simulink model "PendulumSimulation"  (R2020b)
settings: Solver=VariableStepAuto  StartTime=0.0  StopTime=T  RelTol=1e-3
values from neighbouring files (symbols this model uses):
  K = place(A', C', [-5,-2])'./d    [DifferentiatorParameter.m]    (also in Observer_parameter.m = lqr(A, B, eye(4), 10); Project.m = lqr(A, B, eye(4), 2))
  pendulumParameter = PendulumParameter()    [Project.m]
  T = 10    [DifferentiatorParameter.m]    (also in Observer_parameter.m; Project.m)
  Te = 1e-3    (= 0.001)    [DifferentiatorParameter.m]    (also in Observer_parameter.m; Project.m)
  X_eq = [0;pi;0;0]    [Observer_parameter.m]    (also in Project.m = [0;-pi;0;0])
undefined symbols (not defined in the file or in its folder): sigbuilder_block
libraries: simulink_extras x1, vrlib x1
settings Model: Creator=vorps  LastModifiedBy=vorps
settings SolverCC: ZeroCrossAlgorithm=Adaptive
settings DebuggingCC: IgnoredZcDiagnostic=none

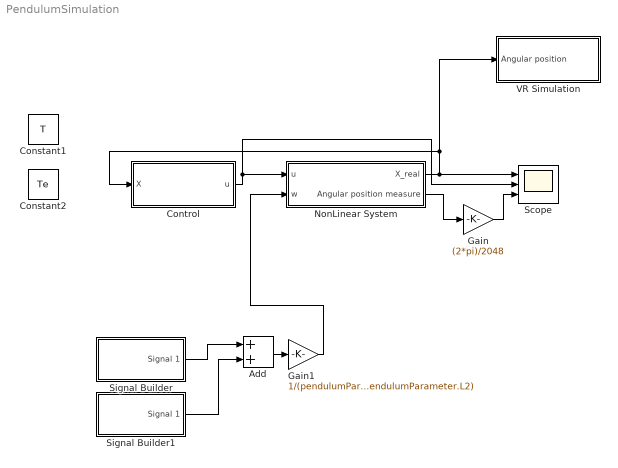
== system PendulumSimulation ==
  Add : Sum
  Constant1 : Constant  Value=T
  Constant2 : Constant  Value=Te
  Control : Subsystem
  Gain : Gain  Gain=(2*pi)/2048
  Gain1 : Gain  Gain=1/(pendulumParameter.M2*pendulumParameter.L2)
  NonLinear System : Subsystem
  Scope : Scope  NumInputPorts=3
  Signal Builder : Subsystem  Tag=STV Subsys  LoadFcn=sigbuilder_block('load');  StartFcn=sigbuilder_block('start');  StopFcn=sigbuilder_block('stop');  ClipboardFcn=sigbuilder_block('clipboard');  mask(Sigbuilder block){tuvar=[0:10]}
      mask help: Simulink:masks:SigbuilderBlock_MD
      mask init:
      | if ~strcmp(get_param(bdroot(gcbh),'SimulationStatus'),'stopped') tuvar = sigbuilder_block('maskInit'); end
      settings: CopyFcn=sigbuilder_block('copy');  DeleteFcn=sigbuilder_block('delete');  ModelCloseFcn=sigbuilder_block('modelClose');  PreSaveFcn=sigbuilder_block('preSave');  PauseFcn=sigbuilder_block('pause');  ContinueFcn=sigbuilder_block('continue');  NameChangeFcn=sigbuilder_block('namechange');  OpenFcn=sigbuilder_block('open',[886.5 189.75 550.5 358.5 ]);  CloseFcn=sigbuilder_block('close');
      mask Display: plot(0, 0, 100, 100,[2, 2, 32, 32, 2], [68, 8, 8, 68, 68],[32, 2], [38, 38], [32, 19, 2],[53, 60, 44], [32, 17, 17, 2],[16, 16, 31, 31]);txt = getActiveGroup(gcbh);text(2, 100, txt,'verticalAlignment', 'top');
  Signal Builder1 : Subsystem  Tag=STV Subsys  LoadFcn=sigbuilder_block('load');  StartFcn=sigbuilder_block('start');  StopFcn=sigbuilder_block('stop');  ClipboardFcn=sigbuilder_block('clipboard');  mask(Sigbuilder block){tuvar=[0:10]}
      mask help: Simulink:masks:SigbuilderBlock_MD
      mask init:
      | if ~strcmp(get_param(bdroot(gcbh),'SimulationStatus'),'stopped') tuvar = sigbuilder_block('maskInit'); end
      settings: CopyFcn=sigbuilder_block('copy');  DeleteFcn=sigbuilder_block('delete');  ModelCloseFcn=sigbuilder_block('modelClose');  PreSaveFcn=sigbuilder_block('preSave');  PauseFcn=sigbuilder_block('pause');  ContinueFcn=sigbuilder_block('continue');  NameChangeFcn=sigbuilder_block('namechange');  OpenFcn=sigbuilder_block('open',[846.75 188.25 544.5 355.5 ]);  CloseFcn=sigbuilder_block('close');
      mask Display: plot(0, 0, 100, 100,[2, 2, 32, 32, 2], [68, 8, 8, 68, 68],[32, 2], [38, 38], [32, 19, 2],[53, 60, 44], [32, 17, 17, 2],[16, 16, 31, 31]);txt = getActiveGroup(gcbh);text(2, 100, txt,'verticalAlignment', 'top');
  VR Simulation : Subsystem
  wires:
  NonLinear System/2(Angular position measure) -> Gain/1
  NonLinear System/1(X_real) -> VR Simulation/1(Angular position), Control/1(X), Scope/1
  Gain1/1 -> NonLinear System/2(w)
  Add/1 -> Gain1/1
  Signal Builder1/1(Signal 1) -> Add/2
  Signal Builder/1(Signal 1) -> Add/1
  Control/1(u) -> Scope/2, NonLinear System/1(u)
  Gain/1 -> Scope/3

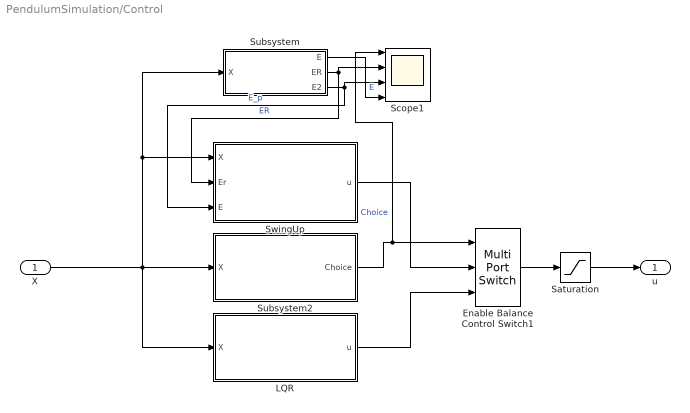
== system PendulumSimulation/Control ==
  X : Inport
  Enable Balance Control Switch1 : MultiPortSwitch  DataPortOrder=Zero-based contiguous  Inputs=2  zeroidx=on
  LQR : Subsystem
  Saturation : Saturate  UpperLimit=10  LowerLimit=-10
  Scope1 : Scope  NumInputPorts=4
  Subsystem : Subsystem
  Subsystem2 : Subsystem
  SwingUp : Subsystem
  u : Outport
  wires:
  LQR/1(u) -> Enable Balance Control Switch1/3
  Subsystem/2(ER) -> SwingUp/2(Er), Scope1/2  "ER"
  SwingUp/1(u) -> Enable Balance Control Switch1/2
  Subsystem/3(E2) -> SwingUp/3(E), Scope1/3  "E_p"
  X/1 -> Subsystem/1(X), SwingUp/1(X), Subsystem2/1(X), LQR/1(X)
  Subsystem2/1(Choice) -> Scope1/1, Enable Balance Control Switch1/1  "Choice"
  Enable Balance Control Switch1/1 -> Saturation/1
  Saturation/1 -> u/1
  Subsystem/1(E) -> Scope1/4  "E"

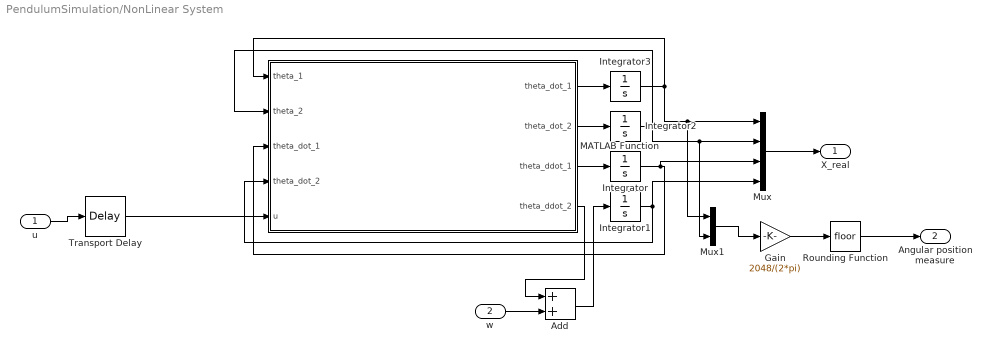
== system PendulumSimulation/NonLinear System ==
  u : Inport
  w : Inport  Port=2
  Add : Sum
  Gain : Gain  Gain=2048/(2*pi)
  Integrator : Integrator
  Integrator1 : Integrator
  Integrator2 : Integrator  InitialCondition=0.1
  Integrator3 : Integrator
  MATLAB Function : MATLAB Function  TreatAsAtomicUnit=on
  Mux : Mux
  Mux1 : Mux  Inputs=2
  Rounding Function : Rounding
  Transport Delay : TransportDelay  DelayTime=0.02
  X_real : Outport
  Angular position measure : Outport  Port=2
  wires:
  Mux/1 -> X_real/1
  Integrator3/1 -> MATLAB Function/1(theta_1), Mux/1, Mux1/1
  Integrator1/1 -> MATLAB Function/4("theta_dot_2 "), Mux/4
  Integrator2/1 -> MATLAB Function/2(theta_2), Mux1/2, Mux/2
  Integrator/1 -> Mux/3, MATLAB Function/3("theta_dot_1 ")
  MATLAB Function/3(theta_ddot_1) -> Integrator/1
  MATLAB Function/1(theta_dot_1) -> Integrator3/1
  Transport Delay/1 -> MATLAB Function/5(u)
  Gain/1 -> Rounding Function/1
  Rounding Function/1 -> Angular position measure/1
  Mux1/1 -> Gain/1
  w/1 -> Add/2
  MATLAB Function/2(theta_dot_2) -> Integrator2/1
  MATLAB Function/4(theta_ddot_2) -> Add/1
  Add/1 -> Integrator1/1
  u/1 -> Transport Delay/1

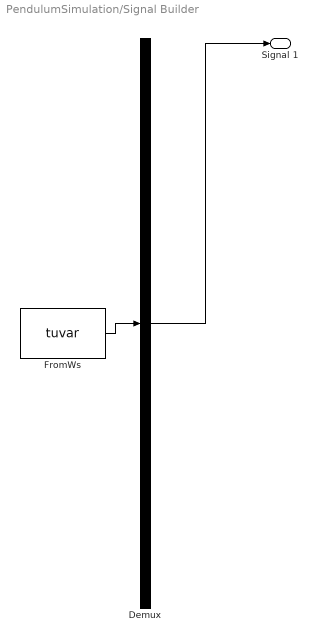
== system PendulumSimulation/Signal Builder ==
  Demux : Demux  Tag=STV Demux  Outputs=1
      settings: DisplayOption=none
  FromWs : FromWorkspace  Tag=STV FromWs  VariableName=tuvar
      SigBuilderData=|
      | common.afterFinalStr = 'Extrapolate'
      | common.sampleTime = 0
      | dataSet.timeRange = [0 10]
      | dataSet.name = 'Group 1'
      | sbobj.Groups.Name = 'Group 1'
      | sbobj.Groups.Signals.Name = 'Signal 1'
      | sbobj.Groups.Signals.XData = [0 4 4.2 4.2 10]
      | sbobj.Groups.Signals.YData = [0 0 0.2 0 0]
  Signal 1 : Outport  Tag=STV Outport
  wires:
  Demux/1 -> Signal 1/1
  FromWs/1 -> Demux/1

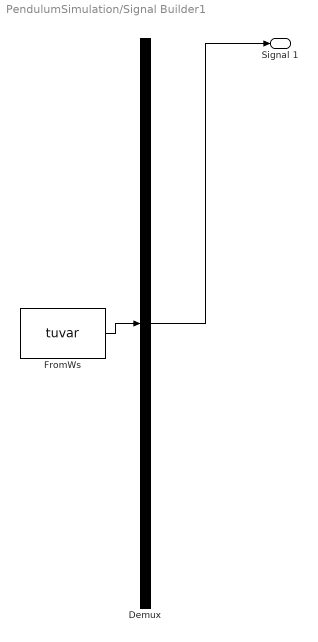
== system PendulumSimulation/Signal Builder1 ==
  Demux : Demux  Tag=STV Demux  Outputs=1
      settings: DisplayOption=none
  FromWs : FromWorkspace  Tag=STV FromWs  VariableName=tuvar
      SigBuilderData=|
      | common.afterFinalStr = 'Extrapolate'
      | common.sampleTime = 0
      | dataSet.timeRange = [0 10]
      | dataSet.name = 'Group 1'
      | sbobj.Groups.Name = 'Group 1'
      | sbobj.Groups.Signals.Name = 'Signal 1'
      | sbobj.Groups.Signals.XData = [0 6.5 6.7 6.7 10]
      | sbobj.Groups.Signals.YData = [0 0 0.4 0 0]
  Signal 1 : Outport  Tag=STV Outport
  wires:
  Demux/1 -> Signal 1/1
  FromWs/1 -> Demux/1

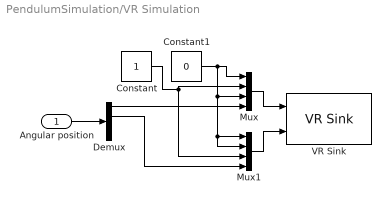
== system PendulumSimulation/VR Simulation ==
  Angular position : Inport
  Constant : Constant
  Constant1 : Constant  Value=0
  Demux : Demux
  Mux : Mux
  Mux1 : Mux
  VR Sink : vrlib/VR Sink  InstantiateOnLoad=on  SampleTime=-1  ViewEnable=on  RemoteChange=off  RemoteView=off  FieldsWritten=Rotary_Arm.rotation.4.1.1.double#Pendulum.rotation.4.1.1.double  WorldFileName=/home/vorps/Documents/Etude/M2/Projet/Modelling/Pendulum.x3d  AutoView=off  VideoDimensions=[]  AllowVariableSize=off
  wires:
  Constant1/1 -> Mux1/2, Mux1/1, Mux/3, Mux/1
  Demux/1 -> Mux/4
  Mux1/1 -> VR Sink/2
  Mux/1 -> VR Sink/1
  Constant/1 -> Mux1/3, Mux/2
  Angular position/1 -> Demux/1
  Demux/2 -> Mux1/4

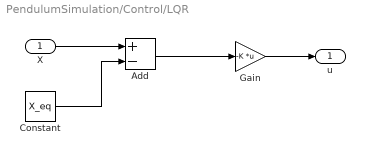
== system PendulumSimulation/Control/LQR ==
  X : Inport
  Add : Sum  Inputs=+-
  Constant : Constant  Value=X_eq
  Gain : Gain  Gain=-K  Multiplication=Matrix(K*u)
  u : Outport
  wires:
  Add/1 -> Gain/1
  Constant/1 -> Add/2
  Gain/1 -> u/1
  X/1 -> Add/1

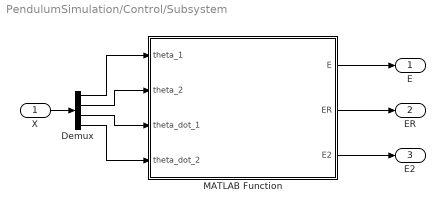
== system PendulumSimulation/Control/Subsystem ==
  X : Inport
  Demux : Demux
  MATLAB Function : MATLAB Function  TreatAsAtomicUnit=on
  E : Outport
  ER : Outport  Port=2
  E2 : Outport  Port=3
  wires:
  X/1 -> Demux/1
  Demux/1 -> MATLAB Function/1(theta_1)
  Demux/2 -> MATLAB Function/2(theta_2)
  Demux/3 -> MATLAB Function/3(theta_dot_1)
  Demux/4 -> MATLAB Function/4(theta_dot_2)
  MATLAB Function/1(E) -> E/1
  MATLAB Function/2(ER) -> ER/1
  MATLAB Function/3(E2) -> E2/1

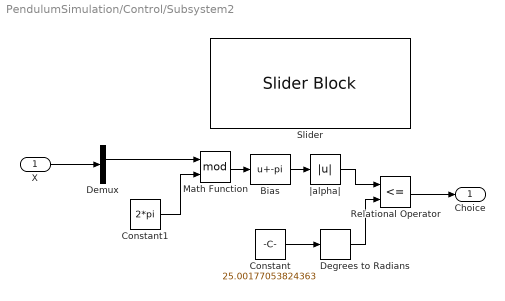
== system PendulumSimulation/Control/Subsystem2 ==
  X : Inport
  Bias : Bias  Bias=-pi
  Constant : Constant  Value=25.00177053824363
  Constant1 : Constant  Value=2*pi
  Degrees to Radians : simulink_extras/Transformations/Degrees to Radians
  Demux : Demux
  Math Function : Math  Operator=mod  SignedPower=on  SaturateOnIntegerOverflow=on
  Relational Operator : RelationalOperator  Operator=<=  OutDataTypeStr=boolean  RndMeth=Simplest
  Slider : SliderBlock  ScaleMax=180
  |alpha| : Abs
  Choice : Outport
  wires:
  X/1 -> Demux/1
  Math Function/1 -> Bias/1
  Demux/2 -> Math Function/1
  Relational Operator/1 -> Choice/1
  Constant1/1 -> Math Function/2
  Bias/1 -> |alpha|/1
  |alpha|/1 -> Relational Operator/1
  Constant/1 -> Degrees to Radians/1
  Degrees to Radians/1 -> Relational Operator/2

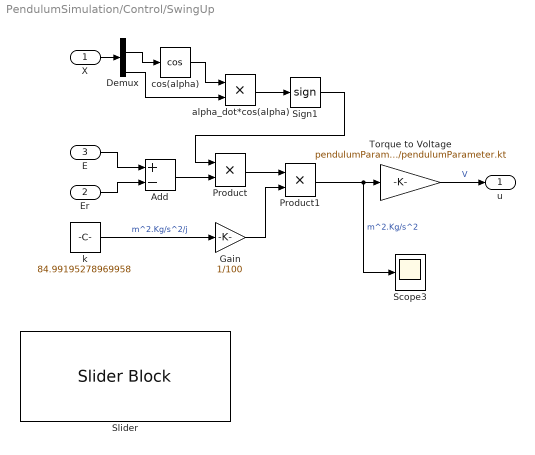
== system PendulumSimulation/Control/SwingUp ==
  X : Inport
  Er : Inport  Port=2
  E : Inport  Port=3
  Add : Sum  Inputs=+-
  Demux : Demux
  Gain : Gain  Gain=1/100
  Product : Product
  Product1 : Product
  Scope3 : Scope
  Sign1 : Signum  ZeroCross=off
  Slider : SliderBlock
  Torque to Voltage : Gain  Gain=pendulumParameter.Rm/pendulumParameter.kt
  alpha_dot*cos(alpha) : Product  RndMeth=Zero
  cos(alpha) : Trigonometry  Operator=cos
  k : Constant  Value=84.99195278969958
  u : Outport  VectorParamsAs1DForOutWhenUnconnected=off
  wires:
  X/1 -> Demux/1
  E/1 -> Add/1
  Er/1 -> Add/2
  cos(alpha)/1 -> alpha_dot*cos(alpha)/1
  Demux/2 -> cos(alpha)/1
  alpha_dot*cos(alpha)/1 -> Sign1/1
  Product/1 -> Product1/1
  k/1 -> Gain/1  "m^2.Kg/s^2/j"
  Demux/4 -> alpha_dot*cos(alpha)/2
  Product1/1 -> Scope3/1, Torque to Voltage/1  "m^2.Kg/s^2"
  Torque to Voltage/1 -> u/1  "V"
  Sign1/1 -> Product/1
  Add/1 -> Product/2
  Gain/1 -> Product1/2

== matlab function PendulumSimulation/Control/Subsystem/MATLAB Function ==
  data: theta_1 input; E output; theta_2 input; theta_dot_1 input; theta_dot_2 input; ER output; E2 output
function [E, ER, E2]  = energie(theta_1, theta_2, theta_dot_1, theta_dot_2)
    coder.extrinsic('evalin');
    pp = PendulumParameter();
    pp = evalin('base','pendulumParameter'); 
    E_p1 = 0;
    E_p2 = pp.g*pp.M2*pp.L2*(1-cos(theta_2))/2;
    E_k1 = 1/2*pp.J1*theta_dot_1^2;
    E_k2 = 1/2*theta_dot_1^2*(pp.M2*pp.L2^2+pp.J2*sin(theta_2)^2)+1/2*theta_dot_2^2*pp.J2 +pp.M2*pp.L1*pp.L2/2*cos(theta_2)*theta_dot_1*theta_dot_2;
    E = E_p1+E_p2+E_k1+E_k2;
    ER =pp.g*pp.M2*pp.L2;
    E2 = E_p2+theta_dot_2^2*pp.J2/2;
end

== matlab function PendulumSimulation/NonLinear System/MATLAB Function ==
  data: theta_1 input; theta_2 input; theta_dot_1 input; theta_dot_2 input; u input; theta_dot_1 output; theta_dot_2 output; theta_ddot_1 output; theta_ddot_2 output
function [theta_dot_1,theta_dot_2,theta_ddot_1,theta_ddot_2]=PendulumNonLinearModel_internal(theta_1,theta_2,theta_dot_1,theta_dot_2,u)
    coder.extrinsic('evalin');
    pp = PendulumParameter();
    pp = evalin('base','pendulumParameter');
    [theta_dot_1,theta_dot_2,theta_ddot_1,theta_ddot_2]=PendulumNonLinearModel(pp, theta_1,theta_2,theta_dot_1,theta_dot_2,u);
end
